simulink model "Validation_sim"  (R2026a)
settings: Solver=VariableStepAuto  StopTime=2500
settings Model: Creator=20251791  LastModifiedBy=20251791

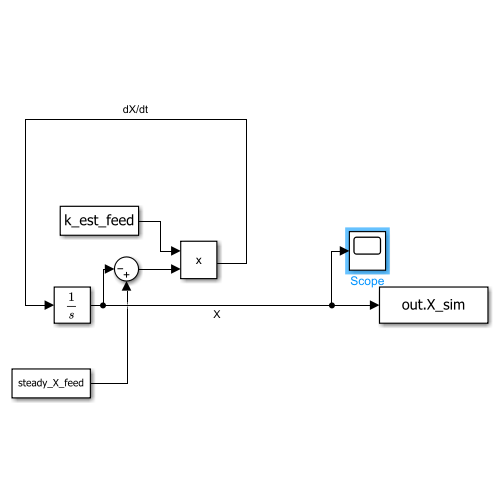
[thumbnail: Simulink's stored preview of the top-level diagram]
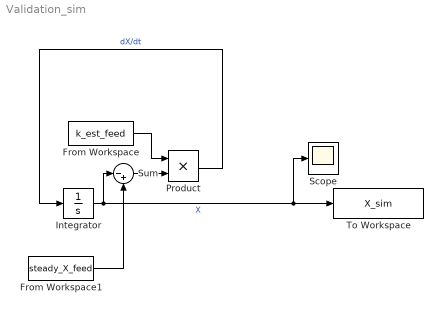
== system Validation_sim ==
  From Workspace : FromWorkspace  VariableName=k_est_feed
  From Workspace1 : FromWorkspace  VariableName=steady_X_feed
  Integrator : Integrator  InitialCondition=0.4
  Product : Product
  Scope : Scope
      settings: ActiveDisplayYMinimum=-0.13901574895897617  ActiveDisplayYMaximum=0.68581270244977377
  Sum : Sum  Inputs=|-+
  To Workspace : ToWorkspace  VariableName=X_sim  SaveFormat=Timeseries  SampleTime=-1
  wires:
  Integrator/1 -> To Workspace/1, Scope/1, Sum/1  "X"
  From Workspace1/1 -> Sum/2
  Sum/1 -> Product/2
  From Workspace/1 -> Product/1
  Product/1 -> Integrator/1  "dX/dt"
